simulink model "encoder_quadratura"  (R2012b)
settings: Solver=ode3  StartTime=0.0  StopTime=3  FixedStep=1e-4  RelTol=1e-6
settings Model: Creator=Juliano  LastModifiedBy=Juliano

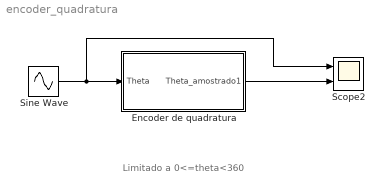
== system encoder_quadratura ==
  note: Limitado a 0<=theta<360
  Encoder de quadratura : Subsystem  mask{Nr=72}
      mask prompts: Nr "Número de pulsos por revolução"
  Scope2 : Scope  NumInputPorts=2
      settings: ShowLegends=on  YMin=150~0  YMax=575~375
  Sine Wave : Sin  Amplitude=360  SampleTime=0
  wires:
  Sine Wave/1 -> Scope2/1, Encoder de quadratura/1(Theta)
  Encoder de quadratura/1(Theta_amostrado1) -> Scope2/2

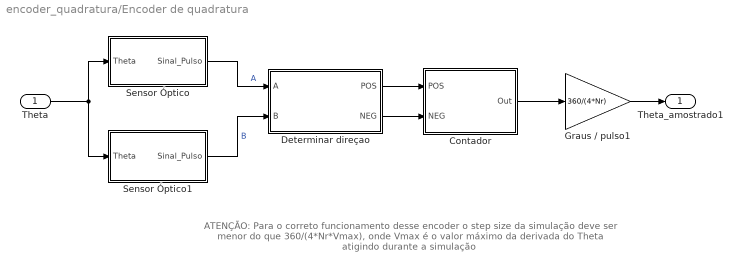
== system encoder_quadratura/Encoder de quadratura ==
  note: ATENÇÃO: Para o correto funcionamento desse encoder o step size da simulação deve ser menor do que 360/(4*Nr*Vmax),
      | onde Vmax é o valor máximo da derivada do Theta atigindo durante a simulação
  Theta : Inport
  Contador : Subsystem
  Determinar direçao : Subsystem
  Graus / pulso1 : Gain  Gain=360/(4*Nr)
  Sensor Óptico : Subsystem
  Sensor Óptico1 : Subsystem
  Theta_amostrado1 : Outport
  wires:
  Theta/1 -> Sensor Óptico1/1(Theta), Sensor Óptico/1(Theta)
  Sensor Óptico/1(Sinal_Pulso) -> Determinar direçao/1(A)  "A"
  Sensor Óptico1/1(Sinal_Pulso) -> Determinar direçao/2(B)  "B"
  Determinar direçao/1(POS) -> Contador/1(POS)
  Determinar direçao/2(NEG) -> Contador/2(NEG)
  Contador/1(Out) -> Graus / pulso1/1
  Graus / pulso1/1 -> Theta_amostrado1/1

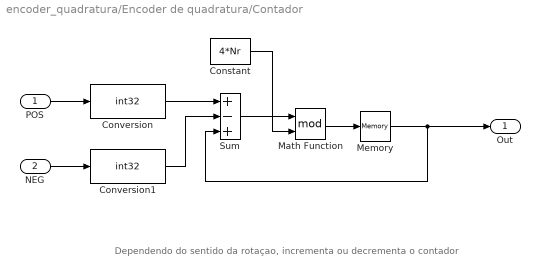
== system encoder_quadratura/Encoder de quadratura/Contador ==
  note: Dependendo do sentido da rotaçao, incrementa ou decrementa o contador
  POS : Inport
  NEG : Inport  Port=2
  Constant : Constant  Value=4*Nr
  Conversion : DataTypeConversion  OutDataTypeStr=int32
  Conversion1 : DataTypeConversion  OutDataTypeStr=int32
  Math Function : Math  Operator=mod  SaturateOnIntegerOverflow=on
  Memory : Memory
  Sum : Sum  Inputs=+-+
  Out : Outport
  wires:
  Sum/1 -> Math Function/1
  Memory/1 -> Out/1, Sum/3
  Math Function/1 -> Memory/1
  POS/1 -> Conversion/1
  Conversion/1 -> Sum/1
  Conversion1/1 -> Sum/2
  NEG/1 -> Conversion1/1
  Constant/1 -> Math Function/2

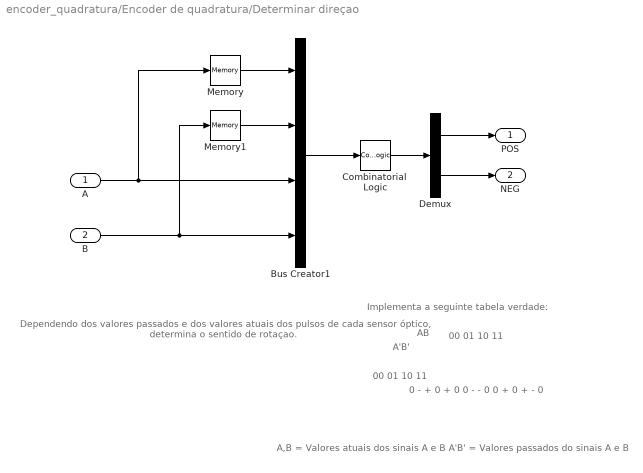
== system encoder_quadratura/Encoder de quadratura/Determinar direçao ==
  note: A,B = Valores atuais dos sinais A e B
      | A'B' = Valores passados do sinais A e B
  note: A'B'
  note: AB
  note: Implementa a seguinte tabela verdade:
  note: 0	-	+	0
      | +	0	0	-
      | -	0	0	+
      | 0	+	-	0
  note: 00 01 10 11
  note: 00
      | 01
      | 10
      | 11
  note: Dependendo dos valores passados e dos valores atuais
      | dos pulsos de cada sensor óptico, determina o sentido
      | de rotaçao.
  A : Inport
  B : Inport  Port=2
  Bus Creator1 : BusCreator
  Combinatorial  Logic : CombinatorialLogic  TruthTable=[ 0 0 ; 0 1 ; 1 0 ; 0 0 ; 1 0 ; 0 0 ; 0 0 ; 0 1 ; 0 1 ; 0 0 ; 0 0 ; 1 0 ; 0 0 ; 1 0 ; 0 1 ; 0 0]
  Demux : Demux  Outputs=2
  Memory : Memory
  Memory1 : Memory
  POS : Outport
  NEG : Outport  Port=2
  wires:
  Demux/1 -> POS/1
  A/1 -> Memory/1, Bus Creator1/3
  Demux/2 -> NEG/1
  Combinatorial  Logic/1 -> Demux/1
  Memory/1 -> Bus Creator1/1
  Bus Creator1/1 -> Combinatorial  Logic/1
  Memory1/1 -> Bus Creator1/2
  B/1 -> Memory1/1, Bus Creator1/4

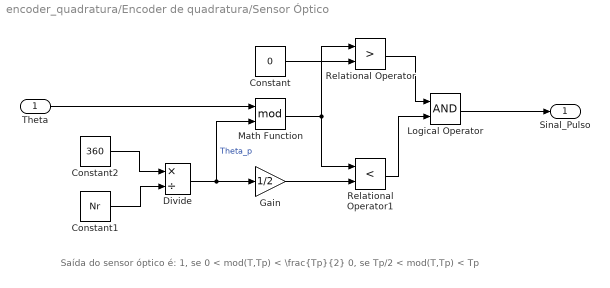
== system encoder_quadratura/Encoder de quadratura/Sensor Óptico ==
  note: Saída do sensor óptico é:
      | 1, se	0 < mod(T,Tp) < \frac{Tp}{2}
      |  0, se      Tp/2 < mod(T,Tp) < Tp
  Theta : Inport
  Constant : Constant  Value=0
  Constant1 : Constant  Value=Nr
  Constant2 : Constant  Value=360
  Divide : Product  Inputs=*/
  Gain : Gain  Gain=1/2
  Logical Operator : Logic  AllPortsSameDT=off  OutDataTypeStr=boolean
  Math Function : Math  Operator=mod  SaturateOnIntegerOverflow=on
  Relational Operator : RelationalOperator  Operator=>  OutDataTypeStr=boolean
  Relational Operator1 : RelationalOperator  Operator=<  OutDataTypeStr=boolean
  Sinal_Pulso : Outport
  wires:
  Math Function/1 -> Relational Operator1/1, Relational Operator/1
  Theta/1 -> Math Function/1
  Relational Operator/1 -> Logical Operator/1
  Relational Operator1/1 -> Logical Operator/2
  Constant/1 -> Relational Operator/2
  Divide/1 -> Math Function/2, Gain/1  "Theta_p"
  Gain/1 -> Relational Operator1/2
  Logical Operator/1 -> Sinal_Pulso/1
  Constant2/1 -> Divide/1
  Constant1/1 -> Divide/2

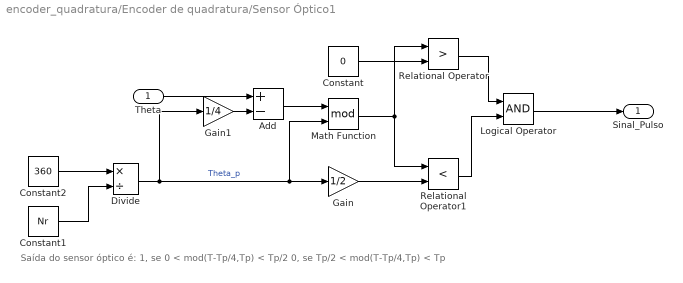
== system encoder_quadratura/Encoder de quadratura/Sensor Óptico1 ==
  note: Saída do sensor óptico é:
      | 1, se	0 < mod(T-Tp/4,Tp) < Tp/2
      |  0, se     Tp/2 < mod(T-Tp/4,Tp) < Tp
  Theta : Inport
  Add : Sum  Inputs=+-
  Constant : Constant  Value=0
  Constant1 : Constant  Value=Nr
  Constant2 : Constant  Value=360
  Divide : Product  Inputs=*/
  Gain : Gain  Gain=1/2
  Gain1 : Gain  Gain=1/4
  Logical Operator : Logic  AllPortsSameDT=off  OutDataTypeStr=boolean
  Math Function : Math  Operator=mod  SaturateOnIntegerOverflow=on
  Relational Operator : RelationalOperator  Operator=>  OutDataTypeStr=boolean
  Relational Operator1 : RelationalOperator  Operator=<  OutDataTypeStr=boolean
  Sinal_Pulso : Outport
  wires:
  Constant1/1 -> Divide/2
  Constant2/1 -> Divide/1
  Logical Operator/1 -> Sinal_Pulso/1
  Gain/1 -> Relational Operator1/2
  Divide/1 -> Gain1/1, Gain/1, Math Function/2  "Theta_p"
  Constant/1 -> Relational Operator/2
  Relational Operator1/1 -> Logical Operator/2
  Relational Operator/1 -> Logical Operator/1
  Math Function/1 -> Relational Operator/1, Relational Operator1/1
  Add/1 -> Math Function/1
  Theta/1 -> Add/1
  Gain1/1 -> Add/2
